simulink model "ProyectoGlobal_AyCD_Cantu_LagoTejo_OPCUA"  (R2021a)
settings: Solver=ode23  StartTime=0.0  StopTime=inf  MinStep=1e-4
undefined symbols (not defined in the file): a_hMax, a_tMax, b_cx, b_cy, b_eq_h, b_eq_t, b_hb, b_hEb, b_t, b_tb, b_tw, b_wu, bah, bat, bcx, bcy, CI_h, CI_t, Cond_Ini_h, Cond_Ini_t, g, H_c, i_h, i_t, k_cy, k_tw, k_wu, Kcy, Kd_bal, Kp_bal, ksah, ksat, ksiah, ksiat, lim_xDer, lim_xDer_ult, lim_xIzq, lim_xIzq_ult, lim_yInf, lim_yInf_ult, lim_ySup, lim_ySup_ult, M_cMax, M_cMin, M_eq_h, M_eq_t, M_s, M_t, r_hd, r_td, T_hbMax, T_hEbMax, T_hmMax, T_tbMax, T_tmMax, tau_hm, tau_tm, v_hMax_0, v_tMax, xc ... (+2)
libraries: simulink x13, opclib x3
(part 1 of 3)
settings Model: SimulationMode=accelerator  Creator=Maxi  LastModifiedBy=maxim
settings SolverCC: InitialStep=1e-3  MaxConsecutiveZCs=10000  MaxConsecutiveMinStep=10000000  ZeroCrossAlgorithm=Adaptive  AlgebraicLoopSolver=TrustRegion
settings DebuggingCC: AlgebraicLoopMsg=none  MaskedZcDiagnostic=none  IgnoredZcDiagnostic=none  SFUnusedDataAndEventsDiag=none  UnderSpecifiedDimensionMsg=warning
settings RTWCC: DLArmComputeVersion=20.02.1

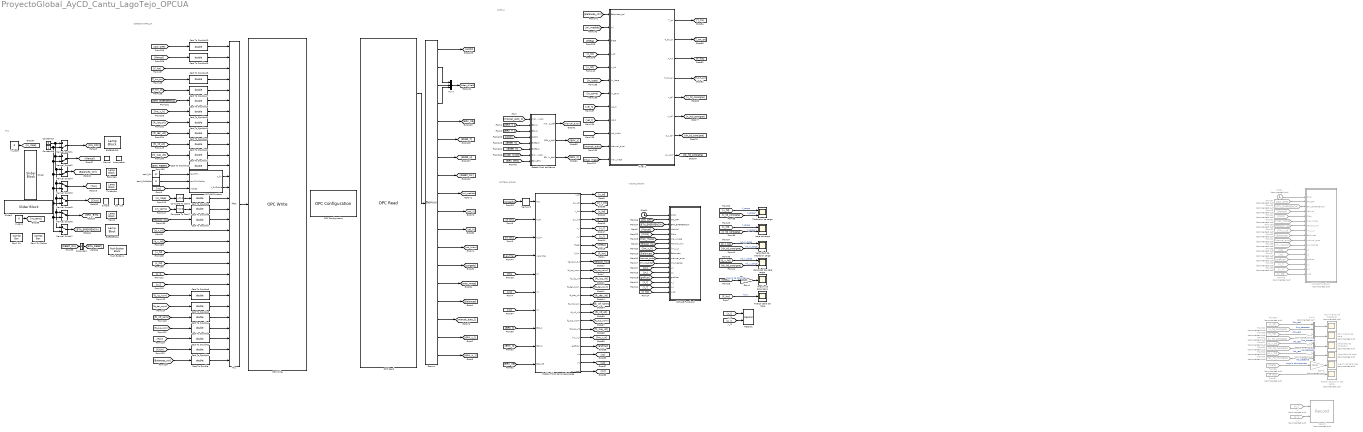
== system ProyectoGlobal_AyCD_Cantu_LagoTejo_OPCUA ==
  note: CODESYS-OPC_UA
  note: HMI
  note: VISUALIZACION
  note: SISTEMA FÍSICO
  note: NIVEL 2
  "  Do" : LampBlock  LabelPosition=Hide
  Angulo de balanceo : Scope  Commented=on
  Angulo de balanceo1 : Scope
  Automático : LampBlock  LabelPosition=Hide
  Balanceo : LampBlock  LabelPosition=Hide
  Carril Fin : ComboBox  LabelPosition=Hide  SelectedLabel=17
      settings: Values={{'1', '2', '3', '4', '5', '6', '7', '8', '9', '10', '11', '12', '13', '14', '15', '16', '17', '18'}, [1 2 3 4 5 6 7 8 9 10 11 12 13 14 15 16 17 18]}
  Carril Fin Doble : ComboBox  LabelPosition=Hide  SelectedLabel=5
      settings: Values={{'1', '2', '3', '4', '5', '6', '7', '8', '9', '10', '11', '12', '13', '14', '15', '16', '17', '18'}, [1 2 3 4 5 6 7 8 9 10 11 12 13 14 15 16 17 18]}
  Cast To Double{,1..20} (21 alike) : DataTypeConversion  OutDataTypeStr=double
  Clock : Clock  Commented=on
  Clock1 : Clock
  Compare To Zero2 : simulink/Logic and Bit Operations/Compare To Zero  relop=~=  OutDataTypeStr=boolean
  Compare To Zero7 : simulink/Logic and Bit Operations/Compare To Zero  relop=~=  OutDataTypeStr=boolean
  Constant17 : Constant  Value=0
  Constant18 : Constant
  Demux : Demux  Outputs=18
  EMERGENCIA : LampBlock  LabelPosition=Hide
  ENCENDIDO : LampBlock  LabelPosition=Hide
  Estado Final de Frenos : Subsystem
  Frenos : LampBlock  LabelPosition=Hide
  From105 : From  Commented=on  GotoTag=Tension_hw
  From13 : From  Commented=on  GotoTag=Manual
  From21 : From  Commented=on  GotoTag=manual_auto
  From38 : From  Commented=on  GotoTag=x_l
  From39 : From  Commented=on  GotoTag=y_l
  From45 : From  Commented=on  GotoTag=x_td
  From53 : From  Commented=on  GotoTag=Balanceo
  From57 : From  Commented=on  GotoTag=yc
  From58 : From  Commented=on  GotoTag=ml_medida
  From59 : From  Commented=on  GotoTag=graficar
  From61 : From  Commented=on  GotoTag=max_masa
  From63 : From  Commented=on  GotoTag=lim_v_h
  From64 : From  Commented=on  GotoTag=Ciclo
  From66 : From  Commented=on  GotoTag=BTN_EMERGENCIA
  From67 : From  Commented=on  GotoTag=ON_OFF
  From85 : From  Commented=on  GotoTag=xc
  From86 : From  Commented=on  GotoTag=theta
  From87 : From  Commented=on  GotoTag=F_hw
  From88 : From  Commented=on  GotoTag=x_hd
  From89 : From  Commented=on  GotoTag=x_td
  From90 : From  Commented=on  GotoTag=x_td_consigna
  From91 : From  Commented=on  GotoTag=x_hd_consigna
  From92 : From  Commented=on  GotoTag=d_x_td
  From93 : From  Commented=on  GotoTag=d_x_hd
  From94 : From  Commented=on  GotoTag=dx_hd_consigna
  From95 : From  Commented=on  GotoTag=dx_td_consigna
  Fuerza cable de izaje : Scope
  Fuerza de tension del cable : Scope  Commented=on
  Gain1 : Gain  Gain=180/pi
  Gain3 : Gain  Commented=on  Gain=180/pi
  Izaje de carga : Scope  NumInputPorts=2
  MATLAB Function : MATLAB Function  TreatAsAtomicUnit=on
  MATLAB Function1 : MATLAB Function  Commented=on  TreatAsAtomicUnit=on
  MATLAB Function2 : MATLAB Function  TreatAsAtomicUnit=on
  Manual : LampBlock  LabelPosition=Hide
  Manual Switch1 : ManualSwitch  CurrentSetting=0
  Manual Switch2 : ManualSwitch  CurrentSetting=0
  Manual Switch{3,5..7} (4 alike) : ManualSwitch
  Manual Switch4 : ManualSwitch  CurrentSetting=0
  Memory5 : Memory
  Modelo Fisico Carro-Izaje-Carga : Subsystem
  Movimiento de Izaje : Scope  Commented=on
  Movimiento de Traslacion : Scope  Commented=on
  Mux : Mux  Inputs=30
  Mux{1..4} (4 alike) : Mux  Commented=on  Inputs=2
  Mux7 : Mux  Inputs=3
  Nivel 2 : Subsystem
  OPC Configuration : opclib/OPC Configuration  opcServers=localhost/CoDeSys.OPC.DA/10  errMissingItems=Error  errReadWrite=Warn  errShutdown=Error  errRTViolation=Warn  rtEnable=on  speedup=1  showLatency=off  beingUsed=on
      settings: SourceProductBaseCode=OT
  OPC Read : opclib/OPC Read  serverHost=localhost  serverID=CoDeSys.OPC.DA  itemIDs=PLC1.Application.GVL.sistOK, PLC1.Application.GVL.manual_auto_N0, PLC1.Application.GVL.BRK_t_N0, PLC1.Application.GVL.BRK_h_N0, PLC1.Application.GVL.BRK_hE, PLC1.Application.GVL.EMER_t, PLC1.Application.GVL.EMER_h, PLC1.Application.GVL.RESET_OK, PLC1.Application.GVL.m_l_calc, PLC1.Application.GVL.vel_t, PLC1.Application.GVL.vel_h, PLC1.Application.GVL.vel_hMax, PLC1.Application.GVL.cargado, PLC1.Application.GVL.max_masa, PLC1.Application.GVL.Balanceo, PLC1.Application.GVL.manual_auto_N1, PLC1.Application.GVL.BRK_t_N1, PLC1.Application.GVL.BRK_h_N1  readMode=Synchronous (cache)  dataType=double  updateRate=0.5  showQual=on  showTS=on  tsMode=Seconds since start
      settings: SourceProductBaseCode=OT
  OPC Write : opclib/OPC Write  serverHost=localhost  serverID=CoDeSys.OPC.DA  itemIDs=PLC1.Application.GVL.ON_OFF, PLC1.Application.GVL.Manual, PLC1.Application.GVL.F_hw, PLC1.Application.GVL.T_hm_on, PLC1.Application.GVL.T_tm_on, PLC1.Application.GVL.BTN_EMERGENCIA, PLC1.Application.GVL.lim_v_h, PLC1.Application.GVL.fc_izq_ult, PLC1.Application.GVL.fc_der_ult, PLC1.Application.GVL.fc_inf_ult, PLC1.Application.GVL.fc_sup_ult, PLC1.Application.GVL.BTN_RESET, PLC1.Application.GVL.X_fin, PLC1.Application.GVL.X_finDoble, PLC1.Application.GVL.in_izaje_on, PLC1.Application.GVL.in_carro_on, PLC1.Application.GVL.Tension_hw, PLC1.Application.GVL.d_x_td, PLC1.Application.GVL.d_x_h, PLC1.Application.GVL.x_td, PLC1.Application.GVL.x_h, PLC1.Application.GVL.x_l, PLC1.Application.GVL.y_l, PLC1.Application.GVL.fc_izq_norm, PLC1.Application.GVL.fc_der_norm, PLC1.Application.GVL.fc_inf_norm, PLC1.Application.GVL.fc_sup_norm, PLC1.Application.GVL.TLK, PLC1.Application.GVL.Ciclo_Doble, PLC1.Application.GVL.Balanceo_ctrl  writeMode=Synchronous  updateRate=0
      settings: SourceProductBaseCode=OT
  Push Button1 : PushButtonBlock  ButtonText=RESET
  Record : Record  Commented=on  FileSettingsInternal="{\"entries\":[{\"content\":{\"excelSettings\":{\"content\":{},\"type\":\"Streamout.ExcelSettings\"}},\"type\":\"Streamout.FileSettingStorage\",\"uuid\":\"83574828-c938-4f10-812a-cc88b85f0559\"}],\"packageUris\":[\"http://schema.mathworks.com/mf0/streamout_blocks/R2020a\"],\"version\":\"1.0\"}"  Layout=[1 1]  SignalsInternal="{\"entries\":[{\"content\":{\"signals\":[{\"content\":{\"blockPath\":[\"ProyectoGlobal_AyCD_Cantu_LagoTejo_OPCUA/Record\"],\"channel\":[],\"dimensions\":[1],\"domain\":\"proyectoglobal_aycd_cantu_lagotejo_opcua/record\",\"lineColor\":\"#edb120\",\"plots\":[1],\"port\":1,\"sid\":[],\"signalID\":143384,\"signalName\":\"x_l\"},\"type\":\"RecordBlkView.Signal\",\"uuid\":\"7d16d182-9664-43c6-b73f-e6d938bfe76a\"},{\"content\":{\"blockPath\":[\"ProyectoGlobal_AyCD_Cantu_LagoTejo_OPCUA/Record\"],\"channel\":[],\"dimensions\":[1],\"domain\":\"proyectoglobal_aycd_cantu_lagotejo_opcua/record\",\"lineColor\":\"#7e2f8e\",\"plots\":[1],\"port\":2,\"sid\":[],\"signalID\":143387,\"signalName\":\"y_l\"},\"type\":\"RecordBlkView.Signal\",\"uuid\":\"076d3fa6-6312-4b84-8d5b-4d468d9208bc\"},{\"content\":{\"blockPath\":[\"ProyectoGlobal_AyCD_Cantu_LagoTejo_OPCUA/Record\"],\"channel\":[],\"dimensions\":[1,32],\"domain\":\"proyectoglobal_aycd_cantu_lagotejo_opcua/record\",\"hasChildren\":true,\"lineColor\":\"#77ac30\",\"plots\":[],\"port\":3,\"sid\":[],\"signalID\":143390,\"signalName\":\"x_perfil\"},\"type\":\"RecordBlkView.Signal\",\"uuid\":\"d0347f4d-14fa-415f-80ee-b1275109c274\"},{\"content\":{\"blockPath\":[\"ProyectoGlobal_AyCD_Cantu_LagoTejo_OPCUA/Record\"],\"channel\":[1,1],\"dimensions\":[1,32],\"domain\":\"proyectoglobal_aycd_cantu_lagotejo_opcua/record\",\"lineColor\":\"#4dbeee\",\"parentID\":143390,\"plots\":[1],\"port\":3,\"sid\":[],\"signalID\":143391,\"signalName\":\"x_perfil\"},\"type\":\"RecordBlkView.Signal\",\"uuid\":\"956556d7-e2bf-48ab-9849-fbb8e8c5bf0b\"},{\"content\":{\"blockPath\":[\"ProyectoGlobal_AyCD_Cantu_LagoTejo_OPCUA/Record\"],\"channel\":[1,2],\"dimensions\":[1,32],\"domain\":\"proyectoglobal_aycd_cantu_lagotejo_opcua/record\",\"lineColor\":\"#fe330a\",\"parentID\":143390,\"plots\":[1],\"port\":3,\"sid\":[],\"signalID\":143392,\"signalName\":\"x_perfil\"},\"type\":\"RecordBlkView.Signal\",\"uuid\":\"90f3ee63-8a15-4922-9693-af30819c6b68\"},{\"content\":{\"blockPath\":[\"ProyectoGlobal_AyCD_Cantu_LagoTejo_OPCUA/Record\"],\"channel\":[1,3],\"dimensions\":[1,32],\"domain\":\"proyectoglobal_aycd_cantu_lagotejo_opcua/record\",\"lineColor\":\"#22b573\",\"parentID\":143390,\"plots\":[],\"port\":3,\"sid\":[],\"signalID\":143393,\"signalName\":\"x_perfil\"},\"type\":\"RecordBlkView.Signal\",\"uuid\":\"0737fd52-0f8e-4f07-9be5-7340ac8ab493\"},{\"content\":{\"blockPath\":[\"ProyectoGlobal_AyCD_Cantu_LagoTejo_OPCUA/Record\"],\"channel\":[1,4],\"dimensions\":[1,32],\"domain\":\"proyectoglobal_aycd_cantu_lagotejo_opcua/record\",\"lineColor\":\"#0072bd\",\"parentID\":143390,\"plots\":[],\"port\":3,\"sid\":[],\"signalID\":143394,\"signalName\":\"x_perfil\"},\"type\":\"RecordBlkView.Signal\",\"uuid\":\"eaa2f601-4cab-45bc-af26-de2e9a567bc7\"},{\"content\":{\"blockPath\":[\"ProyectoGlobal_AyCD_Cantu_LagoTejo_OPCUA/Record\"],\"channel\":[1,5],\"dimensions\":[1,32],\"domain\":\"proyectoglobal_aycd_cantu_lagotejo_opcua/record\",\"lineColor\":\"#d95319\",\"parentID\":143390,\"plots\":[],\"port\":3,\"sid\":[],\"signalID\":143395,\"signalName\":\"x_perfil\"},\"type\":\"RecordBlkView.Signal\",\"uuid\":\"e999367c-c6e6-47ae-8ef4-1182ecbbac9a\"},{\"content\":{\"blockPath\":[\"ProyectoGlobal_AyCD_Cantu_LagoTejo_OPCUA/Record\"],\"channel\":[1,6],\"dimensions\":[1,32],\"domain\":\"proyectoglobal_aycd_cantu_lagotejo_opcua/record\",\"lineColor\":\"#edb120\",\"parentID\":143390,\"plots\":[],\"port\":3,\"sid\":[],\"signalID\":143396,\"signalName\":\"x_perfil\"},\"type\":\"RecordBlkView.Signal\",\"uuid\":\"d576ea24-b850-4519-8fe0-3fd5bf825d31\"},{\"content\":{\"blockPath\":[\"ProyectoGlobal_AyCD_Cantu_LagoTejo_OPCUA/Record\"],\"channel\":[1,7],\"dimensions\":[1,32],\"domain\":\"proyectoglobal_aycd_cantu_lagotejo_opcua/record\",\"lineColor\":\"#7e2f8e\",\"parentID\":143390,\"plots\":[],\"port\":3,\"sid\":[],\"signalID\":143397,\"signalName\":\"x_perfil\"},\"type\":\"RecordBlkView.Signal\",\"uuid\":\"6768b15a-231d-4f71-8817-07cc83716bdf\"},{\"content\":{\"blockPath\":[\"ProyectoGlobal_AyCD_Cantu_LagoTejo_OPCUA/Record\"],\"channel\":[1,8],\"dimensions\":[1,32],\"domain\":\"proyectoglobal_aycd_cantu_lagotejo_opcua/record\",\"lineColor\":\"#77ac30\",\"parentID\":143390,\"plots\":[],\"port\":3,\"sid\":[],\"signalID\":143398,\"signalName\":\"x_perfil\"},\"type\":\"RecordBlkView.Signal\",\"uuid\":\"5aca1eef-53df-4844-8a6f-1da2cede1d1f\"},{\"content\":{\"blockPath\":[\"ProyectoGlobal_AyCD_Cantu_LagoTejo_OPCUA/Record\"],\"channel\":[1,9],\"dimensions\":[1,32],\"domain\":\"proyectoglobal_aycd_cantu_lagotejo_opcua/record\",\"lineColor\":\"#4dbeee\",\"parentID\":143390,\"plots\":[],\"port\":3,\"sid\":[],\"signalID\":143399,\"signalName\":\"x_perfil\"},\"type\":\"RecordBlkView.Signal\",\"uuid\":\"df343d5e-4161-4a59-8c86-37a0bed5a69e\"},{\"content\":{\"blockPath\":[\"ProyectoGlobal_AyCD_Cantu_LagoTejo_OPCUA/Record\"],\"channel\":[1,10],\"dimensions\":[1,32],\"domain\":\"proyectoglobal_aycd_cantu_lagotejo_opcua/record\",\"lineColor\":\"#a2142f\",\"parentID\":143390,\"plots\":[],\"port\":3,\"sid\":[],\"signalID\":143400,\"signalName\":\"x_perfil\"},\"type\":\"RecordBlkView.Signal\",\"uuid\":\"c0d71ad5-ff15-447b-8560-7dbe90ebf72c\"},{\"content\":{\"blockPath\":[\"ProyectoGlobal_AyCD_Cantu_LagoTejo_OPCUA/Record\"],\"channel\":[1,11],\"dimensions\":[1,32],\"domain\":\"proyectoglobal_aycd_cantu_lagotejo_opcua/record\",\"lineColor\":\"#139fff\",\"parentID\":143390,\"plots\":[],\"port\":3,\"sid\":[],\"signalID\":143401,\"signalName\":\"x_perfil\"},\"type\":\"RecordBlkView.Signal\",\"uuid\":\"414505d4-3ae9-4320-b8df-a821bdfefbb2\"},{\"content\":{\"blockPath\":[\"ProyectoGlobal_AyCD_Cantu_LagoTejo_OPCUA/Record\"],\"channel\":[1,12],\"dimensions\":[1,32],\"domain\":\"proyectoglobal_aycd_cantu_lagotejo_opcua/record\",\"lineColor\":\"#ff6929\",\"parentID\":143390,\"plots\":[],\"port\":3,\"sid\":[],\"signalID\":143402,\"signalName\":\"x_perfil\"},\"type\":\"RecordBlkView.Signal\",\"uuid\":\"31229263-3321-4b0d-b4da-0e2665f6cea7\"},{\"content\":{\"blockPath\":[\"ProyectoGlobal_AyCD_Cantu_LagoTejo_OPCUA/Record\"],\"channel\":[1,13],\"dimensions\":[1,32],\"domain\":\"proyectoglobal_aycd_cantu_lagotejo_opcua/record\",\"lineColor\":\"#b746ff\",\"parentID\":143390,\"plots\":[],\"port\":3,\"sid\":[],\"signalID\":143403,\"signalName\":\"x_perfil\"},\"type\":\"RecordBlkView.Signal\",\"uuid\":\"7159e0c8-8d8e-406a-9ea1-5bf641c6b7f4\"},{\"content\":{\"blockPath\":[\"ProyectoGlobal_AyCD_Cantu_LagoTejo_OPCUA/Record\"],\"channel\":[1,14],\"dimensions\":[1,32],\"domain\":\"proyectoglobal_aycd_cantu_lagotejo_opcua/record\",\"lineColor\":\"#64d413\",\"parentID\":143390,\"plots\":[],\"port\":3,\"sid\":[],\"signalID\":143404,\"signalName\":\"x_perfil\"},\"type\":\"RecordBlkView.Signal\",\"uuid\":\"d7101733-b8cc-452e-b2de-7163db0d39dd\"},{\"content\":{\"blockPath\":[\"ProyectoGlobal_AyCD_Cantu_LagoTejo_OPCUA/Record\"],\"channel\":[1,15],\"dimensions\":[1,32],\"domain\":\"proyectoglobal_aycd_cantu_lagotejo_opcua/record\",\"lineColor\":\"#ff13a6\",\"parentID\":143390,\"plots\":[],\"port\":3,\"sid\":[],\"signalID\":143405,\"signalName\":\"x_perfil\"},\"type\":\"RecordBlkView.Signal\",\"uuid\":\"24b40f8c-9900-4ead-bb14-ddf082488a3a\"},{\"content\":{\"blockPath\":[\"ProyectoGlobal_AyCD_Cantu_LagoTejo_OPCUA/Record\"],\"channel\":[1,16],\"dimensions\":[1,32],\"domain\":\"proyectoglobal_aycd_cantu_lagotejo_opcua/record\",\"lineColor\":\"#fe330a\",\"parentID\":143390,\"plots\":[],\"port\":3,\"sid\":[],\"signalID\":143406,\"signalName\":\"x_perfil\"},\"type\":\"RecordBlkView.Signal\",\"uuid\":\"1591ce88-9e53-41fd-af70-3c081883c238\"},{\"content\":{\"blockPath\":[\"ProyectoGlobal_AyCD_Cantu_LagoTejo_OPCUA/Record\"],\"channel\":[1,17],\"dimensions\":[1,32],\"domain\":\"proyectoglobal_aycd_cantu_lagotejo_opcua/record\",\"lineColor\":\"#22b573\",\"parentID\":143390,\"plots\":[],\"port\":3,\"sid\":[],\"signalID\":143407,\"signalName\":\"x_perfil\"},\"type\":\"RecordBlkView.Signal\",\"uuid\":\"10fe3ff4-922a-443a-ac8c-dc8104dc2ff4\"},{\"content\":{\"blockPath\":[\"ProyectoGlobal_AyCD_Cantu_LagoTejo_OPCUA/Record\"],\"channel\":[1,18],\"dimensions\":[1,32],\"domain\":\"proyectoglobal_aycd_cantu_lagotejo_opcua/record\",\"lineColor\":\"#0072bd\",\"parentID\":143390,\"plots\":[],\"port\":3,\"sid\":[],\"signalID\":143408,\"signalName\":\"x_perfil\"},\"type\":\"RecordBlkView.Signal\",\"uuid\":\"4ff0454d-2fab-4ca4-b881-5e21ff589f9a\"},{\"content\":{\"blockPath\":[\"ProyectoGlobal_AyCD_Cantu_LagoTejo_OPCUA/Record\"],\"channel\":[1,19],\"dimensions\":[1,32],\"domain\":\"proyectoglobal_aycd_cantu_lagotejo_opcua/record\",\"lineColor\":\"#d95319\",\"parentID\":143390,\"plots\":[],\"port\":3,\"sid\":[],\"signalID\":143409,\"signalName\":\"x_perfil\"},\"type\":\"RecordBlkView.Signal\",\"uuid\":\"5c85a36e-d81b-41d2-b86d-f6d12f36d804\"},{\"content\":{\"blockPath\":[\"ProyectoGlobal_AyCD_Cantu_LagoTejo_OPCUA/Record\"],\"channel\":[1,20],\"dimensions\":[1,32],\"domain\":\"proyectoglobal_aycd_cantu_lagotejo_opcua/record\",\"lineColor\":\"#edb120\",\"parentID\":143390,\"plots\":[],\"port\":3,\"sid\":[],\"signalID\":143410,\"signalName\":\"x_perfil\"},\"type\":\"RecordBlkView.Signal\",\"uuid\":\"173f3093-86c6-4463-8a83-77c99f06a859\"},{\"content\":{\"blockPath\":[\"ProyectoGlobal_AyCD_Cantu_LagoTejo_OPCUA/Record\"],\"channel\":[1,21],\"dimensions\":[1,32],\"domain\":\"proyectoglobal_aycd_cantu_lagotejo_opcua/record\",\"lineColor\":\"#7e2f8e\",\"parentID\":143390,\"plots\":[],\"port\":3,\"sid\":[],\"signalID\":143411,\"signalName\":\"x_perfil\"},\"type\":\"RecordBlkView.Signal\",\"uuid\":\"e8e81720-94e5-44e4-996f-40043cf66178\"},{\"content\":{\"blockPath\":[\"ProyectoGlobal_AyCD_Cantu_LagoTejo_OPCUA/Record\"],\"channel\":[1,22],\"dimensions\":[1,32],\"domain\":\"proyectoglobal_aycd_cantu_lagotejo_opcua/record\",\"lineColor\":\"#77ac30\",\"parentID\":143390,\"plots\":[],\"port\":3,\"sid\":[],\"signalID\":143412,\"signalName\":\"x_perfil\"},\"type\":\"RecordBlkView.Signal\",\"uuid\":\"8f6c6ccf-cadd-4e1a-b9a5-523af91b5fa9\"},{\"content\":{\"blockPath\":[\"ProyectoGlobal_AyCD_Cantu_LagoTejo_OPCUA/Record\"],\"channel\":[1,23],\"dimensions\":[1,32],\"domain\":\"proyectoglobal_aycd_cantu_lagotejo_opcua/record\",\"lineColor\":\"#4dbeee\",\"parentID\":143390,\"plots\":[],\"port\":3,\"sid\":[],\"signalID\":143413,\"signalName\":\"x_perfil\"},\"type\":\"RecordBlkView.Signal\",\"uuid\":\"97ead022-de46-45e3-a805-1dd7a210c9fb\"},{\"content\":{\"blockPath\":[\"ProyectoGlobal_AyCD_Cantu_LagoTejo_OPCUA/Record\"],\"channel\":[1,24],\"dimensions\":[1,32],\"domain\":\"proyectoglobal_aycd_cantu_lagotejo_opcua/record\",\"lineColor\":\"#a2142f\",\"parentID\":143390,\"plots\":[],\"port\":3,\"sid\":[],\"signalID\":143414,\"signalName\":\"x_perfil\"},\"type\":\"RecordBlkView.Signal\",\"uuid\":\"f84a2c40-5edf-4623-8dc3-e3257f0f3b7c\"},{\"content\":{\"blockPath\":[\"ProyectoGlobal_AyCD_Cantu_LagoTejo_OPCUA/Record\"],\"channel\":[1,25],\"dimensions\":[1,32],\"domain\":\"proyectoglobal_aycd_cantu_lagotejo_opcua/record\",\"lineColor\":\"#139fff\",\"parentID\":143390,\"plots\":[],\"port\":3,\"sid\":[],\"signalID\":143415,\"signalName\":\"x_perfil\"},\"type\":\"RecordBlkView.Signal\",\"uuid\":\"92cfa7cd-7b05-4834-835f-d8ad1141618b\"},{\"content\":{\"blockPath\":[\"ProyectoGlobal_AyCD_Cantu_LagoTejo_OPCUA/Record\"],\"channel\":[1,26],\"dimensions\":[1,32],\"domain\":\"proyectoglobal_aycd_cantu_lagotejo_opcua/record\",\"lineColor\":\"#ff6929\",\"parentID\":143390,\"plots\":[],\"port\":3,\"sid\":[],\"signalID\":143416,\"signalName\":\"x_perfil\"},\"type\":\"RecordBlkView.Signal\",\"uuid\":\"d23a6982-a689-4d8b-be0c-f8f9ed596f6a\"},{\"content\":{\"blockPath\":[\"ProyectoGlobal_AyCD_Cantu_LagoTejo_OPCUA/Record\"],\"channel\":[1,27],\"dimensions\":[1,32],\"domain\":\"proyectoglobal_aycd_cantu_lagotejo_opcua/record\",\"lineColor\":\"#b746ff\",\"parentID\":143390,\"plots\":[],\"port\":3,\"sid\":[],\"signalID\":143417,\"signalName\":\"x_perfil\"},\"type\":\"RecordBlkView.Signal\",\"uuid\":\"258c98dd-eb41-4a98-b7b8-69592a103465\"},{\"content\":{\"blockPath\":[\"ProyectoGlobal_AyCD_Cantu_LagoTejo_OPCUA/Record\"],\"channel\":[1,28],\"dimensions\":[1,32],\"domain\":\"proyectoglobal_aycd_cantu_lagotejo_opcua/record\",\"lineColor\":\"#64d413\",\"parentID\":143390,\"plots\":[],\"port\":3,\"sid\":[],\"signalID\":143418,\"signalName\":\"x_perfil\"},\"type\":\"RecordBlkView.Signal\",\"uuid\":\"48e00f9c-d444-451e-b404-7275da64b877\"},{\"content\":{\"blockPath\":[\"ProyectoGlobal_AyCD_Cantu_LagoTejo_OPCUA/Record\"],\"channel\":[1,29],\"dimensions\":[1,32],\"domain\":\"proyectoglobal_aycd_cantu_lagotejo_opcua/record\",\"lineColor\":\"#ff13a6\",\"parentID\":143390,\"plots\":[],\"port\":3,\"sid\":[],\"signalID\":143419,\"signalName\":\"x_perfil\"},\"type\":\"RecordBlkView.Signal\",\"uuid\":\"f22eb2c5-5226-4c97-b4d0-11799347ecd3\"},{\"content\":{\"blockPath\":[\"ProyectoGlobal_AyCD_Cantu_LagoTejo_OPCUA/Record\"],\"channel\":[1,30],\"dimensions\":[1,32],\"domain\":\"proyectoglobal_aycd_cantu_lagotejo_opcua/record\",\"lineColor\":\"#fe330a\",\"parentID\":143390,\"plots\":[],\"port\":3,\"sid\":[],\"signalID\":143420,\"signalName\":\"x_perfil\"},\"type\":\"RecordBlkView.Signal\",\"uuid\":\"ca7d4a3f-21b7-48bc-b0d3-3a72059f5e6f\"},{\"content\":{\"blockPath\":[\"ProyectoGlobal_AyCD_Cantu_LagoTejo_OPCUA/Record\"],\"channel\":[1,31],\"dimensions\":[1,32],\"domain\":\"proyectoglobal_aycd_cantu_lagotejo_opcua/record\",\"lineColor\":\"#22b573\",\"parentID\":143390,\"plots\":[],\"port\":3,\"sid\":[],\"signalID\":143421,\"signalName\":\"x_perfil\"},\"type\":\"RecordBlkView.Signal\",\"uuid\":\"2834c59d-0ed6-47b6-b74c-7cd6bccee760\"},{\"content\":{\"blockPath\":[\"ProyectoGlobal_AyCD_Cantu_LagoTejo_OPCUA/Record\"],\"channel\":[1,32],\"dimensions\":[1,32],\"domain\":\"proyectoglobal_aycd_cantu_lagotejo_opcua/record\",\"lineColor\":\"#0072bd\",\"parentID\":143390,\"plots\":[],\"port\":3,\"sid\":[],\"signalID\":143422,\"signalName\":\"x_perfil\"},\"type\":\"RecordBlkView.Signal\",\"uuid\":\"3f80176a-175b-4c9b-8b65-0ccab0f2275a\"},{\"content\":{\"blockPath\":[\"ProyectoGlobal_AyCD_Cantu_LagoTejo_OPCUA/Record\"],\"channel\":[],\"dimensions\":[1,32],\"domain\":\"proyectoglobal_aycd_cantu_lagotejo_opcua/record\",\"hasChildren\":true,\"lineColor\":\"#a2142f\",\"plots\":[],\"port\":4,\"sid\":[],\"signalID\":143457,\"signalName\":\"y_perfil\"},\"type\":\"RecordBlkView.Signal\",\"uuid\":\"2b6d1931-4834-4e5d-a076-e35bd244ead6\"},{\"content\":{\"blockPath\":[\"ProyectoGlobal_AyCD_Cantu_LagoTejo_OPCUA/Record\"],\"channel\":[1,1],\"dimensions\":[1,32],\"domain\":\"proyectoglobal_aycd_cantu_lagotejo_opcua/record\",\"lineColor\":\"#139fff\",\"parentID\":143457,\"plots\":[1],\"port\":4,\"sid\":[],\"signalID\":143458,\"signalName\":\"y_perfil\"},\"type\":\"RecordBlkView.Signal\",\"uuid\":\"8f1c1fc6-4740-4843-b791-bd5b5adceac1\"},{\"content\":{\"blockPath\":[\"ProyectoGlobal_AyCD_Cantu_LagoTejo_OPCUA/Record\"],\"channel\":[1,2],\"dimensions\":[1,32],\"domain\":\"proyectoglobal_aycd_cantu_lagotejo_opcua/record\",\"lineColor\":\"#d95319\",\"parentID\":143457,\"plots\":[1],\"port\":4,\"sid\":[],\"signalID\":143459,\"signalName\":\"y_perfil\"},\"type\":\"RecordBlkView.Signal\",\"uuid\":\"5b1401a5-a014-43a1-8357-6afc49d5364e\"},{\"content\":{\"blockPath\":[\"ProyectoGlobal_AyCD_Cantu_LagoTejo_OPCUA/Record\"],\"channel\":[1,3],\"dimensions\":[1,32],\"domain\":\"proyectoglobal_aycd_cantu_lagotejo_opcua/record\",\"lineColor\":\"#edb120\",\"parentID\":143457,\"plots\":[],\"port\":4,\"sid\":[],\"signalID\":143460,\"signalName\":\"y_perfil\"},\"type\":\"RecordBlkView.Signal\",\"uuid\":\"dc5790e6-e127-46e6-9f91-486df376b843\"},{\"content\":{\"blockPath\":[\"ProyectoGlobal_AyCD_Cantu_LagoTejo_OPCUA/Record\"],\"channel\":[1,4],\"dimensions\":[1,32],\"domain\":\"proyectoglobal_aycd_cantu_lagotejo_opcua/record\",\"lineColor\":\"#7e2f8e\",\"parentID\":143457,\"plots\":[],\"port\":4,\"sid\":[],\"signalID\":143461,\"signalName\":\"y_perfil\"},\"type\":\"RecordBlkView.Signal\",\"uuid\":\"b6846bb3-c8a4-4935-b723-f56350e6f3e7\"},{\"content\":{\"blockPath\":[\"ProyectoGlobal_AyCD_Cantu_LagoTejo_OPCUA/Record\"],\"channel\":[1,5],\"dimensions\":[1,32],\"domain\":\"proyectoglobal_aycd_cantu_lagotejo_opcua/record\",\"lineColor\":\"#77ac30\",\"parentID\":143457,\"plots\":[],\"port\":4,\"sid\":[],\"signalID\":143462,\"signalName\":\"y_perfil\"},\"type\":\"RecordBlkView.Signal\",\"uuid\":\"61778b0a-d6d5-4fd1-af7d-552c46a7b739\"},{\"content\":{\"blockPath\":[\"ProyectoGlobal_AyCD_Cantu_LagoTejo_OPCUA/Record\"],\"channel\":[1,6],\"dimensions\":[1,32],\"domain\":\"proyectoglobal_aycd_cantu_lagotejo_opcua/record\",\"lineColor\":\"#4dbeee\",\"parentID\":143457,\"plots\":[],\"port\":4,\"sid\":[],\"signalID\":143463,\"signalName\":\"y_perfil\"},\"type\":\"RecordBlkView.Signal\",\"uuid\":\"88f249c5-4b48-4dcd-ba17-0602820ba8a5\"},{\"content\":{\"blockPath\":[\"ProyectoGlobal_AyCD_Cantu_LagoTejo_OPCUA/Record\"],\"channel\":[1,7],\"dimensions\":[1,32],\"domain\":\"proyectoglobal_aycd_cantu_lagotejo_opcua/record\",\"lineColor\":\"#a2142f\",\"parentID\":143457,\"plots\":[],\"port\":4,\"sid\":[],\"signalID\":143464,\"signalName\":\"y_perfil\"},\"type\":\"RecordBlkView.Signal\",\"uuid\":\"39037c46-ccc7-4357-bf22-b743b3991f8b\"},{\"content\":{\"blockPath\":[\"ProyectoGlobal_AyCD_Cantu_LagoTejo_OPCUA/Record\"],\"channel\":[1,8],\"dimensions\":[1,32],\"domain\":\"proyectoglobal_aycd_cantu_lagotejo_opcua/record\",\"lineColor\":\"#139fff\",\"parentID\":143457,\"plots\":[],\"port\":4,\"sid\":[],\"signalID\":143465,\"signalName\":\"y_perfil\"},\"type\":\"RecordBlkView.Signal\",\"uuid\":\"9e9d18a3-0b45-4d94-ab0f-8af43b414047\"},{\"content\":{\"blockPath\":[\"ProyectoGlobal_AyCD_Cantu_LagoTejo_OPCUA/Record\"],\"channel\":[1,9],\"dimensions\":[1,32],\"domain\":\"proyectoglobal_aycd_cantu_lagotejo_opcua/record\",\"lineColor\":\"#ff6929\",\"parentID\":143457,\"plots\":[],\"port\":4,\"sid\":[],\"signalID\":143466,\"signalName\":\"y_perfil\"},\"type\":\"RecordBlkView.Signal\",\"uuid\":\"0ac9721a-646e-41d0-86d9-d8f5d36e8e3d\"},{\"content\":{\"blockPath\":[\"ProyectoGlobal_AyCD_Cantu_LagoTejo_OPCUA/Record\"],\"channel\":[1,10],\"dimensions\":[1,32],\"domain\":\"proyectoglobal_aycd_cantu_lagotejo_opcua/record\",\"lineColor\":\"#b746ff\",\"parentID\":143457,\"plots\":[],\"port\":4,\"sid\":[],\"signalID\":143467,\"signalName\":\"y_perfil\"},\"type\":\"RecordBlkView.Signal\",\"uuid\":\"7e05bec0-8696-4961-a9da-7eebc67db628\"},{\"content\":{\"blockPath\":[\"ProyectoGlobal_AyCD_Cantu_LagoTejo_OPCUA/Record\"],\"channel\":[1,11],\"dimensions\":[1,32],\"domain\":\"proyectoglobal_aycd_cantu_lagotejo_opcua/record\",\"lineColor\":\"#64d413\",\"parentID\":143457,\"plots\":[],\"port\":4,\"sid\":[],\"signalID\":143468,\"signalName\":\"y_perfil\"},\"type\":\"RecordBlkView.Signal\",\"uuid\":\"e6e84412-9acd-4382-aef7-95e2cb4f3bfe\"},{\"content\":{\"blockPath\":[\"ProyectoGlobal_AyCD_Cantu_LagoTejo_OPCUA/Record\"],\"channel\":[1,12],\"dimensions\":[1,32],\"domain\":\"proyectoglobal_aycd_cantu_lagotejo_opcua/record\",\"lineColor\":\"#ff13a6\",\"parentID\":143457,\"plots\":[],\"port\":4,\"sid\":[],\"signalID\":143469,\"signalName\":\"y_perfil\"},\"type\":\"RecordBlkView.Signal\",\"uuid\":\"409ef5a3-7ef1-4d09-9741-f1f210409f09\"},{\"content\":{\"blockPath\":[\"ProyectoGlobal_AyCD_Cantu_LagoTejo_OPCUA/Record\"],\"channel\":[1,13],\"dimensions\":[1,32],\"domain\":\"proyectoglobal_aycd_cantu_lagotejo_opcua/record\",\"lineColor\":\"#fe330a\",\"parentID\":143457,\"plots\":[],\"port\":4,\"sid\":[],\"signalID\":143470,\"signalName\":\"y_perfil\"},\"type\":\"RecordBlkView.Signal\",\"uuid\":\"e6d22919-2b52-4e13-8397-dabdf01daca0\"},{\"content\":{\"blockPath\":[\"ProyectoGlobal_AyCD_Cantu_LagoTejo_OPCUA/Record\"],\"channel\":[1,14],\"dimensions\":[1,32],\"domain\":\"proyectoglobal_aycd_cantu_lagotejo_opcua/record\",\"lineColor\":\"#22b573\",\"parentID\":143457,\"plots\":[],\"port\":4,\"sid\":[],\"signalID\":143471,\"signalName\":\"y_perfil\"},\"type\":\"RecordBlkView.Signal\",\"uuid\":\"d8024cb2-8dea-47f0-9244-8532a877d535\"},{\"content\":{\"blockPath\":[\"ProyectoGlobal_AyCD_Cantu_LagoTejo_OPCUA/Record\"],\"channel\":[1,15],\"dimensions\":[1,32],\"domain\":\"proyectoglobal_aycd_cantu_lagotejo_opcua/record\",\"lineColor\":\"#0072bd\",\"parentID\":143457,\"plots\":[],\"port\":4,\"sid\":[],\"signalID\":143472,\"signalName\":\"y_perfil\"},\"type\":\"RecordBlkView.Signal\",\"uuid\":\"bd1df95d-2f4e-4b5c-9bee-03aadae1e6e1\"},{\"content\":{\"blockPath\":[\"ProyectoGlobal_AyCD_Cantu_LagoTejo_OPCUA/Record\"],\"channel\":[1,16],\"dimensions\":[1,32],\"domain\":\"proyectoglobal_aycd_cantu_lagotejo_opcua/record\",\"lineColor\":\"#d95319\",\"parentID\":143457,\"plots\":[],\"port\":4,\"sid\":[],\"signalID\":143473,\"signalName\":\"y_perfil\"},\"type\":\"RecordBlkView.Signal\",\"uuid\":\"546d976e-8545-40dd-9543-eca1c3ffca2a\"},{\"content\":{\"blockPath\":[\"ProyectoGlobal_AyCD_Cantu_LagoTejo_OPCUA/Record\"],\"channel\":[1,17],\"dimensions\":[1,32],\"domain\":\"proyectoglobal_aycd_cantu_lagotejo_opcua/record\",\"lineColor\":\"#edb120\",\"parentID\":143457,\"plots\":[],\"port\":4,\"sid\":[],\"signalID\":143474,\"signalName\":\"y_perfil\"},\"type\":\"RecordBlkView.Signal\",\"uuid\":\"12ee5f58-67ac-4ca1-9ef6-e6fb16d101e4\"},{\"content\":{\"blockPath\":[\"ProyectoGlobal_AyCD_Cantu_LagoTejo_OPCUA/Record\"],\"channel\":[1,18],\"dimensions\":[1,32],\"domain\":\"proyectoglobal_aycd_cantu_lagotejo_opcua/record\",\"lineColor\":\"#7e2f8e\",\"parentID\":143457,\"plots\":[],\"port\":4,\"sid\":[],\"signalID\":143475,\"signalName\":\"y_perfil\"},\"type\":\"RecordBlkView.Signal\",\"uuid\":\"d2105892-ca9c-4dab-9129-b93fc009cb6e\"},{\"content\":{\"blockPath\":[\"ProyectoGlobal_AyCD_Cantu_LagoTejo_OPCUA/Record\"],\"channel\":[1,19],\"dimensions\":[1,32],\"domain\":\"proyectoglobal_aycd_cantu_lagotejo_opcua/record\",\"lineColor\":\"#77ac30\",\"parentID\":143457,\"plots\":[],\"port\":4,\"sid\":[],\"signalID\":143476,\"signalName\":\"y_perfil\"},\"type\":\"RecordBlkView.Signal\",\"uuid\":\"47c48979-b09e-4e99-93cf-1458c9188519\"},{\"content\":{\"blockPath\":[\"ProyectoGlobal_AyCD_Cantu_LagoTejo_OPCUA/Record\"],\"channel\":[1,20],\"dimensions\":[1,32],\"domain\":\"proyectoglobal_aycd_cantu_lagotejo_opcua/record\",\"lineColor\":\"#4dbeee\",\"parentID\":143457,\"plots\":[1],\"port\":4,\"sid\":[],\"signalID\":143477,\"signalName\":\"y_perfil\"},\"type\":\"RecordBlkView.Signal\",\"uuid\":\"41f9c27c-de5b-4d3a-9dea-89fc7061acef\"},{\"content\":{\"blockPath\":[\"ProyectoGlobal_AyCD_Cantu_LagoTejo_OPCUA/Record\"],\"channel\":[1,21],\"dimensions\":[1,32],\"domain\":\"proyectoglobal_aycd_cantu_lagotejo_opcua/record\",\"lineColor\":\"#a2142f\",\"parentID\":143457,\"plots\":[],\"port\":4,\"sid\":[],\"signalID\":143478,\"signalName\":\"y_perfil\"},\"type\":\"RecordBlkView.Signal\",\"uuid\":\"efaf13c1-fe20-4963-98d4-2d1348af0945\"},{\"content\":{\"blockPath\":[\"ProyectoGlobal_AyCD_Cantu_LagoTejo_OPCUA/Record\"],\"channel\":[1,22],\"dimensions\":[1,32],\"domain\":\"proyectoglobal_aycd_cantu_lagotejo_opcua/record\",\"lineColor\":\"#139fff\",\"parentID\":143457,\"plots\":[],\"port\":4,\"sid\":[],\"signalID\":143479,\"signalName\":\"y_perfil\"},\"type\":\"RecordBlkView.Signal\",\"uuid\":\"e897cc40-d6f3-4498-b124-a5598c43429b\"},{\"content\":{\"blockPath\":[\"ProyectoGlobal_AyCD_Cantu_LagoTejo_OPCUA/Record\"],\"channel\":[1,23],\"dimensions\":[1,32],\"domain\":\"proyectoglobal_aycd_cantu_lagotejo_opcua/record\",\"lineColor\":\"#ff6929\",\"parentID\":143457,\"plots\":[],\"port\":4,\"sid\":[],\"signalID\":143480,\"signalName\":\"y_perfil\"},\"type\":\"RecordBlkView.Signal\",\"uuid\":\"3a346875-d0f4-4f1d-b17d-519f758b664c\"},{\"content\":{\"blockPath\":[\"ProyectoGlobal_AyCD_Cantu_LagoTejo_OPCUA/Record\"],\"channel\":[1,24],\"dimensions\":[1,32],\"domain\":\"proyectoglobal_aycd_cantu_lagotejo_opcua/record\",\"lineColor\":\"#b746ff\",\"parentID\":143457,\"plots\":[],\"port\":4,\"sid\":[],\"signalID\":143481,\"signalName\":\"y_perfil\"},\"type\":\"RecordBlkView.Signal\",\"uuid\":\"76bf5b2e-ffcb-4bdd-a270-609649d416e8\"},{\"content\":{\"blockPath\":[\"ProyectoGlobal_AyCD_Cantu_LagoTejo_OPCUA/Record\"],\"channel\":[1,25],\"dimensions\":[1,32],\"domain\":\"proyectoglobal_aycd_cantu_lagotejo_opcua/record\",\"lineColor\":\"#64d413\",\"parentID\":143457,\"plots\":[],\"port\":4,\"sid\":[],\"signalID\":143482,\"signalName\":\"y_perfil\"},\"type\":\"RecordBlkView.Signal\",\"uuid\":\"4f5bf088-5fb6-4a00-85e5-e2197b71f071\"},{\"content\":{\"blockPath\":[\"ProyectoGlobal_AyCD_Cantu_LagoTejo_OPCUA/Record\"],\"channel\":[1,26],\"dimensions\":[1,32],\"domain\":\"proyectoglobal_aycd_cantu_lagotejo_opcua/record\",\"lineColor\":\"#ff13a6\",\"parentID\":143457,\"plots\":[],\"port\":4,\"sid\":[],\"signalID\":143483,\"signalName\":\"y_perfil\"},\"type\":\"RecordBlkView.Signal\",\"uuid\":\"39e30418-4cb1-4327-b79f-28f02c1a5a21\"},{\"content\":{\"blockPath\":[\"ProyectoGlobal_AyCD_Cantu_LagoTejo_OPCUA/Record\"],\"channel\":[1,27],\"dimensions\":[1,32],\"domain\":\"proyectoglobal_aycd_cantu_lagotejo_opcua/record\",\"lineColor\":\"#fe330a\",\"parentID\":143457,\"plots\":[],\"port\":4,\"sid\":[],\"signalID\":143484,\"signalName\":\"y_perfil\"},\"type\":\"RecordBlkView.Signal\",\"uuid\":\"108605f9-0e74-4845-afda-6c8c3fbf9fc5\"},{\"content\":{\"blockPath\":[\"ProyectoGlobal_AyCD_Cantu_LagoTejo_OPCUA/Record\"],\"channel\":[1,28],\"dimensions\":[1,32],\"domain\":\"proyectoglobal_aycd_cantu_lagotejo_opcua/record\",\"lineColor\":\"#22b573\",\"parentID\":143457,\"plots\":[],\"port\":4,\"sid\":[],\"signalID\":143485,\"signalName\":\"y_perfil\"},\"type\":\"RecordBlkView.Signal\",\"uuid\":\"716c56fe-e41c-4e13-a7a8-10bcfb9040b0\"},{\"content\":{\"blockPath\":[\"ProyectoGlobal_AyCD_Cantu_LagoTejo_OPCUA/Record\"],\"channel\":[1,29],\"dimensions\":[1,32],\"domain\":\"proyectoglobal_aycd_cantu_lagotejo_opcua/record\",\"lineColor\":\"#0072bd\",\"parentID\":143457,\"plots\":[],\"port\":4,\"sid\":[],\"signalID\":143486,\"signalName\":\"y_perfil\"},\"type\":\"RecordBlkView.Signal\",\"uuid\":\"e8db83b6-123b-44c7-b781-03f6ca8d4aab\"},{\"content\":{\"blockPath\":[\"ProyectoGlobal_AyCD_Cantu_LagoTejo_OPCUA/Record\"],\"channel\":[1,30],\"dimensions\":[1,32],\"domain\":\"proyectoglobal_aycd_cantu_lagotejo_opcua/record\",\"lineColor\":\"#d95319\",\"parentID\":143457,\"plots\":[],\"port\":4,\"sid\":[],\"signalID\":143487,\"signalName\":\"y_perfil\"},\"type\":\"RecordBlkView.Signal\",\"uuid\":\"8dddb66e-458c-4295-accf-90f3921de3f3\"},{\"content\":{\"blockPath\":[\"ProyectoGlobal_AyCD_Cantu_LagoTejo_OPCUA/Record\"],\"channel\":[1,31],\"dimensions\":[1,32],\"domain\":\"proyectoglobal_aycd_cantu_lagotejo_opcua/record\",\"lineColor\":\"#edb120\",\"parentID\":143457,\"plots\":[],\"port\":4,\"sid\":[],\"signalID\":143488,\"signalName\":\"y_perfil\"},\"type\":\"RecordBlkView.Signal\",\"uuid\":\"1aab923f-154b-4c82-9907-74b0d9d6c087\"},{\"content\":{\"blockPath\":[\"ProyectoGlobal_AyCD_Cantu_LagoTejo_OPCUA/Record\"],\"channel\":[1,32],\"dimensions\":[1,32],\"domain\":\"proyectoglobal_aycd_cantu_lagotejo_opcua/record\",\"lineColor\":\"#7e2f8e\",\"parentID\":143457,\"plots\":[],\"port\":4,\"sid\":[],\"signalID\":143489,\"signalName\":\"y_perfil\"},\"type\":\"RecordBlkView.Signal\",\"uuid\":\"ddfc17ad-b6a5-42e4-8991-23eb111d2ff9\"}]},\"type\":\"RecordBlkView.InputSignals\",\"uuid\":\"60c02c37-2890-4383-8ffd-f79d336a72cb\"}],\"packageUris\":[\"http://schema.mathworks.com/mf0/streamout_blocks/R2020a\"],\"version\":\"1.0\"}"  VisualizationBindings="{\"xyplotplugin\":{\"info\":[{\"series\":[{\"bindingParametersList\":[{\"parameter\":\"X-Axis\",\"signalID\":143384,\"signalName\":\"x_l\"},{\"parameter\":\"Y-Axis\",\"signalID\":143387,\"signalName\":\"y_l\"}],\"seriesID\":213},{\"bindingParametersList\":[{\"parameter\":\"X-Axis\",\"signalID\":143391,\"signalName\":\"x_perfil(1,1)\"},{\"parameter\":\"Y-Axis\",\"signalID\":143458,\"signalName\":\"y_perfil(1,1)\"}],\"seriesID\":320},{\"bindingParametersList\":[{\"parameter\":\"Y-Axis\",\"signalID\":143477,\"signalName\":\"y_perfil(1,20)\"},{\"parameter\":\"X-Axis\",\"signalID\":143477,\"signalName\":\"y_perfil(1,20)\"}],\"seriesID\":767},{\"bindingParametersList\":[{\"parameter\":\"X-Axis\",\"signalID\":143392,\"signalName\":\"x_perfil(1,2)\"},{\"parameter\":\"Y-Axis\",\"signalID\":143459,\"signalName\":\"y_perfil(1,2)\"}],\"seriesID\":639}],\"subplotID\":1}]}}"
  Record1 : Record  FileSettingsInternal="{\"entries\":[{\"content\":{\"excelSettings\":{\"content\":{},\"type\":\"Streamout.ExcelSettings\"}},\"type\":\"Streamout.FileSettingStorage\",\"uuid\":\"3e7b64e0-0ce2-41f3-8a99-b89d649c3767\"}],\"packageUris\":[\"http://schema.mathworks.com/mf0/streamout_blocks/R2020a\"],\"version\":\"1.0\"}"  Layout=[1 1]  SignalsInternal="{\"entries\":[{\"content\":{\"signals\":[{\"content\":{\"blockPath\":[\"ProyectoGlobal_AyCD_Cantu_LagoTejo_OPCUA/Record1\"],\"channel\":[],\"dimensions\":[1],\"domain\":\"proyectoglobal_aycd_cantu_lagotejo_opcua/record1\",\"lineColor\":\"#edb120\",\"plots\":[1],\"port\":1,\"sid\":[],\"signalID\":143376,\"signalName\":\"x_l1\"},\"type\":\"RecordBlkView.Signal\",\"uuid\":\"afc6e062-fac5-424c-a01c-5c1b65c55174\"},{\"content\":{\"blockPath\":[\"ProyectoGlobal_AyCD_Cantu_LagoTejo_OPCUA/Record1\"],\"channel\":[],\"dimensions\":[1],\"domain\":\"proyectoglobal_aycd_cantu_lagotejo_opcua/record1\",\"lineColor\":\"#7e2f8e\",\"plots\":[1],\"port\":2,\"sid\":[],\"signalID\":143379,\"signalName\":\"y_l1\"},\"type\":\"RecordBlkView.Signal\",\"uuid\":\"d31f8ff2-8118-463d-9920-bb53ea1afa0e\"}]},\"type\":\"RecordBlkView.InputSignals\",\"uuid\":\"31ffbdfa-eeb9-45d9-b521-3a19031a059d\"}],\"packageUris\":[\"http://schema.mathworks.com/mf0/streamout_blocks/R2020a\"],\"version\":\"1.0\"}"  VisualizationBindings="{\"xyplotplugin\":{\"info\":[{\"series\":[{\"bindingParametersList\":[{\"parameter\":\"X-Axis\",\"signalID\":143376,\"signalName\":\"x_l1\"},{\"parameter\":\"Y-Axis\",\"signalID\":143379,\"signalName\":\"y_l1\"}],\"seriesID\":213}],\"subplotID\":1}]}}"
  Simple : LampBlock  LabelPosition=Hide
  Slider : SliderBlock  ScaleMin=-3  ScaleMax=3  TickInterval=1
  Slider1 : SliderBlock  ScaleMin=-4  ScaleMax=+4  TickInterval=1
  Subsystem : Subsystem
  Traslacion de carga : Scope  NumInputPorts=2
  Twistlocks : LampBlock  LabelPosition=Hide
  Velocidad de Izaje : Scope  Commented=on
  Velocidad de Traslacion : Scope  Commented=on
  Velocidad de izaje carga : Scope  NumInputPorts=2
  Velocidad de traslacion carga : Scope  NumInputPorts=2
  "ble   " : LampBlock  LabelPosition=Hide
  carril_fin : Constant  Value=17
  carril_finDoble : Constant  Value=5
  in_carro : Constant  Value=0
  in_izaje : Constant  Value=0
  x_l : From  Commented=on  GotoTag=x_l
  y_l : From  Commented=on  GotoTag=y_l
  tag scope: Orden_Nivel0=global, sistOK=global
  wires:
  Modelo Fisico Carro-Izaje-Carga/1(x_td) -> [x_td]
  Modelo Fisico Carro-Izaje-Carga/3(x_hd) -> [x_hd]
  Modelo Fisico Carro-Izaje-Carga/7(theta) -> [theta]
  [yc] -> Modelo Fisico Carro-Izaje-Carga/6(Yc)
  Modelo Fisico Carro-Izaje-Carga/5(x_l) -> [x_l]
  Modelo Fisico Carro-Izaje-Carga/6(y_l) -> [y_l]
  Modelo Fisico Carro-Izaje-Carga/8(F_hw) -> [F_hw]
  Modelo Fisico Carro-Izaje-Carga/2(d_x_td) -> [d_x_td]
  Modelo Fisico Carro-Izaje-Carga/4(d_x_hd) -> [d_x_hd]
  [T_tm] -> Modelo Fisico Carro-Izaje-Carga/2(T_tm)
  [T_hm] -> Modelo Fisico Carro-Izaje-Carga/3(T_hm)
  [ml] -> Modelo Fisico Carro-Izaje-Carga/5(ml)
  From86/1 -> Gain3/1  "Angulo de balanceo"
  From87/1 -> Fuerza de tension del cable/1
  From94/1 -> Mux4/2  "Vel_deseada"
  From92/1 -> Mux3/1  "Vel_real"
  From91/1 -> Mux2/2  "Pos_deseada"
  Mux2/1 -> Movimiento de Izaje/1
  Mux4/1 -> Velocidad de Izaje/1
  From93/1 -> Mux4/1  "Vel_real"
  From89/1 -> Mux1/1  "Pos_real"
  Mux3/1 -> Velocidad de Traslacion/1
  From90/1 -> Mux1/2  "Pos_deseada"
  From88/1 -> Mux2/1  "Pos_real"
  Mux1/1 -> Movimiento de Traslacion/1
  From95/1 -> Mux3/2  "Vel_deseada"
  Gain3/1 -> Angulo de balanceo/1
  [BRK_h] -> Modelo Fisico Carro-Izaje-Carga/9(BRK_h)
  [BRK_hE] -> Modelo Fisico Carro-Izaje-Carga/10(BRK_hE)
  [BRK_t] -> Modelo Fisico Carro-Izaje-Carga/8(BRK_t)
  Modelo Fisico Carro-Izaje-Carga/15(fc_inf_ult) -> [fc_inf_ult]
  Modelo Fisico Carro-Izaje-Carga/18(lim_v_h) -> [lim_v_h]
  [cargado] -> Memory5/1
  Memory5/1 -> Modelo Fisico Carro-Izaje-Carga/1(TLK)
  Modelo Fisico Carro-Izaje-Carga/14(fc_inf_norm) -> [fc_inf_norm]
  Modelo Fisico Carro-Izaje-Carga/17(fc_sup_ult) -> [fc_sup_ult]
  Modelo Fisico Carro-Izaje-Carga/13(fc_der_ult) -> [fc_der_ult]
  Modelo Fisico Carro-Izaje-Carga/10(fc_izq_norm) -> [fc_izq_norm]
  Modelo Fisico Carro-Izaje-Carga/11(fc_izq_ult) -> [fc_izq_ult]
  Modelo Fisico Carro-Izaje-Carga/12(fc_der_norm) -> [fc_der_norm]
  Modelo Fisico Carro-Izaje-Carga/16(fc_sup_norm) -> [fc_sup_norm]
  [xc] -> Modelo Fisico Carro-Izaje-Carga/7(Xc)
  [vel_hMax] -> Modelo Fisico Carro-Izaje-Carga/4(vel_hMax)
  x_l/1 -> Record/1
  y_l/1 -> Record/2
  Modelo Fisico Carro-Izaje-Carga/9(Tension_hw) -> [Tension_hw]
  Estado Final de Frenos/2(BRK_t_def) -> [BRK_t]
  [EMER_H] -> Estado Final de Frenos/6(EMER_h)
  [Orden_Nivel0] -> Estado Final de Frenos/7(Orden_Nivel0)
  Estado Final de Frenos/3(BRK_h_def) -> [BRK_h]
  [EMER_T] -> Estado Final de Frenos/5(EMER_T)
  [sistOK] -> Estado Final de Frenos/4(sistOK)
  Estado Final de Frenos/1(manual_auto_def) -> [manual_auto]
  [ml_medida] -> Nivel 2/2(ml)
  [x_hd] -> Nivel 2/5(x_hd)
  Nivel 2/5(x_td*) -> [x_td_consigna]
  Nivel 2/2(T_tm_on) -> [T_tm_on]
  Nivel 2/4(T_hm_on) -> [T_hm_on]
  [Balanceo_ctrl] -> Nivel 2/1(Balanceo_ctrl)
  Nivel 2/6(x_hd*) -> [x_hd_consigna]
  Nivel 2/8(d_x_hd*) -> [dx_hd_consigna]
  Nivel 2/1(T_tm) -> [T_tm]
  Nivel 2/3(T_hm) -> [T_hm]
  [vel_h] -> Nivel 2/8(vel_h)
  [x_td] -> Nivel 2/4(x_td)
  [in_izaje] -> Nivel 2/6(in_izaje)
  Nivel 2/7(d_x_td*) -> [dx_td_consigna]
  [theta] -> Nivel 2/3(theta)
  [vel_hMax] -> Nivel 2/10(vel_hMax)
  [in_carro] -> Nivel 2/7(in_carro)
  [max_masa] -> Nivel 2/12(max_masa)
  [manual_auto] -> Nivel 2/11(manual_auto)
  [vel_t] -> Nivel 2/9(vel_t)
  [in_carro] -> Compare To Zero7/1
  [in_izaje] -> Compare To Zero2/1
  [T_tm_on] -> Cast To Double17/1
  Demux/8 -> [RESET_OK]
  [T_hm_on] -> Cast To Double18/1
  [fc_izq_ult] -> Cast To Double14/1
  Mux7/1 -> [Orden_Nivel0]
  Demux/3 -> Mux7/2
  [Manual] -> Cast To Double19/1
  [ON_OFF] -> Cast To Double20/1
  Demux/7 -> [EMER_H]
  [fc_der_ult] -> Cast To Double13/1
  Demux/1 -> [sistOK]
  Demux/4 -> Mux7/3
  [BTN_EMERGENCIA] -> Cast To Double16/1
  [lim_v_h] -> Cast To Double15/1
  Demux/2 -> Mux7/1
  Demux/6 -> [EMER_T]
  [fc_inf_ult] -> Cast To Double12/1
  Demux/5 -> [BRK_hE]
  [F_hw] -> Mux/3
  [fc_sup_ult] -> Cast To Double11/1
  Modelo Fisico Carro-Izaje-Carga/19(graficar) -> [graficar]
  Modelo Fisico Carro-Izaje-Carga/20(xc) -> [xc]
  Modelo Fisico Carro-Izaje-Carga/21(yc) -> [yc]
  Modelo Fisico Carro-Izaje-Carga/22(m_l_real) -> [ml]
  [BTN_RESET] -> Cast To Double10/1
  Constant18/1 -> Manual Switch2/2, Manual Switch4/2, Manual Switch3/2, Manual Switch6/2, Manual Switch7/2, Manual Switch5/2, Manual Switch1/2
  Manual Switch4/1 -> [Balanceo_ctrl]
  in_carro/1 -> [in_carro]
  Manual Switch6/1 -> [BRK_BTN]
  Constant17/1 -> Manual Switch2/1, Manual Switch4/1, Manual Switch3/1, Manual Switch6/1, Manual Switch7/1, Manual Switch5/1, Manual Switch1/1
  Manual Switch1/1 -> [ON_OFF]
  Manual Switch5/1 -> [Ciclo]
  in_izaje/1 -> [in_izaje]
  Manual Switch3/1 -> [TLK]
  Subsystem/1(Out1) -> [BTN_RESET]
  Manual Switch2/1 -> [Manual]
  [RESET_OK] -> Subsystem/1(" ")
  Manual Switch7/1 -> [BTN_EMERGENCIA]
  [BRK_BTN] -> Estado Final de Frenos/8(BRK_BTN)
  Clock/1 -> MATLAB Function1/1(clock)
  From67/1 -> MATLAB Function1/2(ON_OFF)
  From66/1 -> MATLAB Function1/3(BTN_EMERGENCIA)
  From13/1 -> MATLAB Function1/4(Manual)
  From64/1 -> MATLAB Function1/5(Ciclo)
  From61/1 -> MATLAB Function1/6(max_masa)
  From105/1 -> MATLAB Function1/7(Tension_hw)
  From63/1 -> MATLAB Function1/8(lim_v_h)
  From53/1 -> MATLAB Function1/9(Balanceo)
  From21/1 -> MATLAB Function1/10(manual_auto)
  From58/1 -> MATLAB Function1/11(ml_medida)
  From85/1 -> MATLAB Function1/12(xc)
  From57/1 -> MATLAB Function1/13(yc)
  From59/1 -> MATLAB Function1/14(graficar)
  From38/1 -> MATLAB Function1/15(x_l)
  From39/1 -> MATLAB Function1/16(y_l)
  From45/1 -> MATLAB Function1/17(x_td)
  [manual_auto_1] -> Estado Final de Frenos/1(manual_auto_Nivel1)
  [BRK_t_1] -> Estado Final de Frenos/2(BRK_t)
  [BRK_h_1] -> Estado Final de Frenos/3(BRK_h)
  OPC Read/1 -> Demux/1
  Demux/9 -> [ml_medida]
  Demux/10 -> [vel_t]
  Demux/11 -> [vel_h]
  Demux/12 -> [vel_hMax]
  Demux/13 -> [cargado]
  Demux/14 -> [max_masa]
  Demux/15 -> [Balanceo]
  Demux/16 -> [manual_auto_1]
  Demux/17 -> [BRK_t_1]
  Demux/18 -> [BRK_h_1]
  [Tension_hw] -> Cast To Double7/1
  [d_x_td] -> Mux/18
  [d_x_hd] -> Mux/19
  [x_td] -> Mux/20
  [x_hd] -> Mux/21
  [y_l] -> Mux/23
  [x_l] -> Mux/22
  [fc_izq_norm] -> Cast To Double6/1
  [fc_der_norm] -> Cast To Double5/1
  [fc_inf_norm] -> Cast To Double4/1
  [fc_sup_norm] -> Cast To Double3/1
  [TLK] -> Cast To Double2/1
  [Ciclo] -> Cast To Double1/1
  [Balanceo_ctrl] -> Cast To Double/1
  Mux/1 -> OPC Write/1
  Compare To Zero2/1 -> Cast To Double9/1
  Compare To Zero7/1 -> Cast To Double8/1
  MATLAB Function/1(X_fin) -> Mux/13
  MATLAB Function/2(X_finDoble) -> Mux/14
  carril_fin/1 -> MATLAB Function/1(carrilFin)
  carril_finDoble/1 -> MATLAB Function/2(carrilFinDoble)
  [xc] -> MATLAB Function/3(Xcarga)
  Cast To Double/1 -> Mux/30
  Cast To Double1/1 -> Mux/29
  Cast To Double2/1 -> Mux/28
  Cast To Double3/1 -> Mux/27
  Cast To Double4/1 -> Mux/26
  Cast To Double5/1 -> Mux/25
  Cast To Double6/1 -> Mux/24
  Cast To Double7/1 -> Mux/17
  Cast To Double8/1 -> Mux/16
  Cast To Double9/1 -> Mux/15
  Cast To Double10/1 -> Mux/12
  Cast To Double11/1 -> Mux/11
  Cast To Double12/1 -> Mux/10
  Cast To Double13/1 -> Mux/9
  Cast To Double14/1 -> Mux/8
  Cast To Double15/1 -> Mux/7
  Cast To Double16/1 -> Mux/6
  Cast To Double17/1 -> Mux/5
  Cast To Double18/1 -> Mux/4
  Cast To Double19/1 -> Mux/2
  Cast To Double20/1 -> Mux/1
  [x_hd] -> Izaje de carga/1  "Y_carga"
  [d_x_hd] -> Velocidad de izaje carga/1  "vel_Y_carga"
  [y_l] -> Record1/2
  [x_td_consigna] -> Traslacion de carga/2  "X_carga*"
  [dx_hd_consigna] -> Velocidad de izaje carga/2  "vel_y_carga*"
  [d_x_td] -> Velocidad de traslacion carga/1  "vel_X_carga"
  Gain1/1 -> Angulo de balanceo1/1
  [x_hd_consigna] -> Izaje de carga/2  "Y_carga*"
  [x_td] -> MATLAB Function2/17(x_td)
  [F_hw] -> Fuerza cable de izaje/1  "F_hw"
  [yc] -> MATLAB Function2/13(yc)
  [graficar] -> MATLAB Function2/14(graficar)
  [x_l] -> MATLAB Function2/15(x_l)
  [Manual] -> MATLAB Function2/4(Manual)
  [y_l] -> MATLAB Function2/16(y_l)
  [xc] -> MATLAB Function2/12(xc)
  [ml_medida] -> MATLAB Function2/11(ml_medida)
  [x_td] -> Traslacion de carga/1  "X_carga"
  [lim_v_h] -> MATLAB Function2/8(lim_v_h)
  [dx_td_consigna] -> Velocidad de traslacion carga/2  "vel_X_carga*"
  [max_masa] -> MATLAB Function2/6(max_masa)
  [Tension_hw] -> MATLAB Function2/7(Tension_hw)
  [manual_auto] -> MATLAB Function2/10(manual_auto)
  [Ciclo] -> MATLAB Function2/5(Ciclo)
  [ON_OFF] -> MATLAB Function2/2(ON_OFF)
  [theta] -> Gain1/1  "Angulo de balanceo"
  [Balanceo] -> MATLAB Function2/9(Balanceo)
  [BTN_EMERGENCIA] -> MATLAB Function2/3(BTN_EMERGENCIA)
  [x_l] -> Record1/1
  Clock1/1 -> MATLAB Function2/1(clock)

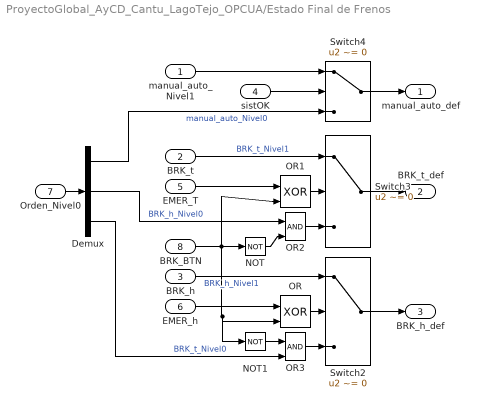
== system ProyectoGlobal_AyCD_Cantu_LagoTejo_OPCUA/Estado Final de Frenos ==
  manual_auto_Nivel1 : Inport
  BRK_t : Inport  Port=2
  BRK_h : Inport  Port=3
  sistOK : Inport  Port=4
  EMER_T : Inport  Port=5
  EMER_h : Inport  Port=6
  Orden_Nivel0 : Inport  Port=7
  BRK_BTN : Inport  Port=8
  Demux : Demux  Outputs=3
  NOT : Logic  Operator=NOT  IconShape=distinctive  AllPortsSameDT=off  OutDataTypeStr=boolean
  NOT1 : Logic  Operator=NOT  IconShape=distinctive  AllPortsSameDT=off  OutDataTypeStr=boolean
  OR : Logic  Operator=XOR  IconShape=distinctive  AllPortsSameDT=off  OutDataTypeStr=boolean
  OR1 : Logic  Operator=XOR  IconShape=distinctive  AllPortsSameDT=off  OutDataTypeStr=boolean
  OR2 : Logic  IconShape=distinctive  AllPortsSameDT=off  OutDataTypeStr=boolean
  OR3 : Logic  IconShape=distinctive  AllPortsSameDT=off  OutDataTypeStr=boolean
  Switch2 : Switch  Criteria=u2 ~= 0
  Switch3 : Switch  Criteria=u2 ~= 0
  Switch4 : Switch  Criteria=u2 ~= 0
  manual_auto_def : Outport
  BRK_t_def : Outport  Port=2
  BRK_h_def : Outport  Port=3
  wires:
  Switch3/1 -> BRK_t_def/1
  Switch2/1 -> BRK_h_def/1
  Switch4/1 -> manual_auto_def/1
  sistOK/1 -> Switch4/2
  BRK_t/1 -> Switch3/1  "BRK_t_Nivel1"
  BRK_h/1 -> Switch2/1  "BRK_h_Nivel1"
  manual_auto_Nivel1/1 -> Switch4/1
  Demux/2 -> OR2/1  "BRK_h_Nivel0"
  Demux/3 -> OR3/2  "BRK_t_Nivel0"
  Orden_Nivel0/1 -> Demux/1
  Demux/1 -> Switch4/3  "manual_auto_Nivel0"
  OR/1 -> Switch2/2
  EMER_T/1 -> OR1/1
  OR1/1 -> Switch3/2
  BRK_BTN/1 -> OR1/2, NOT/1, NOT1/1, OR/2
  OR2/1 -> Switch3/3
  NOT/1 -> OR2/2
  EMER_h/1 -> OR/1
  OR3/1 -> Switch2/3
  NOT1/1 -> OR3/1
